simulink model "simu"  (R2023b)
settings: Solver=VariableStepAuto  StartTime=0.0  StopTime=8  RelTol=1e-3
libraries: simulink x6
settings Model: Creator=denis  LastModifiedBy=andre
settings OptimizationCC: ReuseModelBlockBuffer=off

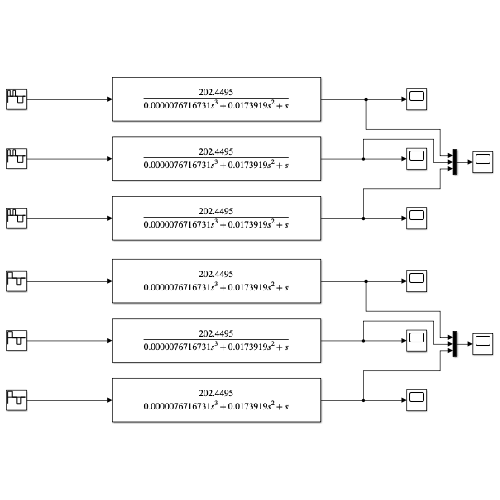
[thumbnail: Simulink's stored preview of the top-level diagram]
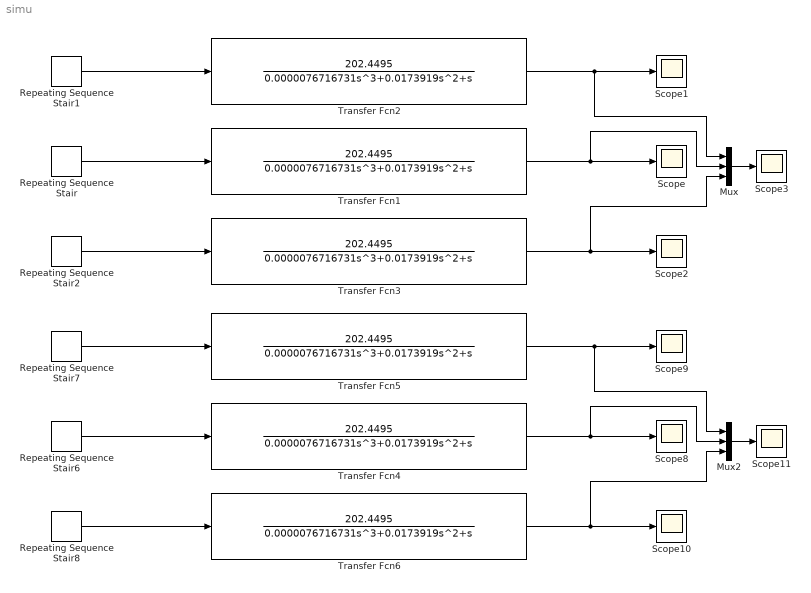
== system simu ==
  Mux : Mux  Inputs=3
  Mux2 : Mux  Inputs=3
  Repeating Sequence Stair : simulink/Sources/Repeating Sequence Stair  OutValues=7.5*[1 0 1 0 -1 -1 0].'  tsamp=1  OutMin=[]  OutMax=[]  OutDataTypeStr=double  OutputDataTypeScalingMode=double  OutDataType=fixdt(0,8)  ConRadixGroup=Best Precision: Vector-wise  OutScaling=2^-12
  Repeating Sequence Stair1 : simulink/Sources/Repeating Sequence Stair  OutValues=9*[1 0 1 0 -1 -1 0].'  tsamp=1  OutMin=[]  OutMax=[]  OutDataTypeStr=double  OutputDataTypeScalingMode=double  OutDataType=fixdt(0,8)  ConRadixGroup=Best Precision: Vector-wise  OutScaling=2^-12
  Repeating Sequence Stair2 : simulink/Sources/Repeating Sequence Stair  OutValues=6*[1 0 1 0 -1 -1 0].'  tsamp=1  OutMin=[]  OutMax=[]  OutDataTypeStr=double  OutputDataTypeScalingMode=double  OutDataType=fixdt(0,8)  ConRadixGroup=Best Precision: Vector-wise  OutScaling=2^-12
  Repeating Sequence Stair6 : simulink/Sources/Repeating Sequence Stair  OutValues=7.5*[1 0 -1 0].'  tsamp=1  OutMin=[]  OutMax=[]  OutDataTypeStr=double  OutputDataTypeScalingMode=double  OutDataType=fixdt(0,8)  ConRadixGroup=Best Precision: Vector-wise  OutScaling=2^-12
  Repeating Sequence Stair7 : simulink/Sources/Repeating Sequence Stair  OutValues=9*[1 0 -1 0].'  tsamp=1  OutMin=[]  OutMax=[]  OutDataTypeStr=double  OutputDataTypeScalingMode=double  OutDataType=fixdt(0,8)  ConRadixGroup=Best Precision: Vector-wise  OutScaling=2^-12
  Repeating Sequence Stair8 : simulink/Sources/Repeating Sequence Stair  OutValues=6*[1 0 -1 0].'  tsamp=1  OutMin=[]  OutMax=[]  OutDataTypeStr=double  OutputDataTypeScalingMode=double  OutDataType=fixdt(0,8)  ConRadixGroup=Best Precision: Vector-wise  OutScaling=2^-12
  Scope{,1..3,8..11} (8 alike) : Scope
  Transfer Fcn{1..6} (6 alike) : TransferFcn  Numerator=[202.4495]  Denominator=[0.0000076716731 0.0173919 1 0]
  wires:
  Repeating Sequence Stair/1 -> Transfer Fcn1/1
  Transfer Fcn1/1 -> Mux/2, Scope/1
  Transfer Fcn2/1 -> Mux/1, Scope1/1
  Repeating Sequence Stair1/1 -> Transfer Fcn2/1
  Transfer Fcn3/1 -> Mux/3, Scope2/1
  Repeating Sequence Stair2/1 -> Transfer Fcn3/1
  Mux/1 -> Scope3/1
  Mux2/1 -> Scope11/1
  Transfer Fcn5/1 -> Mux2/1, Scope9/1
  Transfer Fcn6/1 -> Mux2/3, Scope10/1
  Transfer Fcn4/1 -> Mux2/2, Scope8/1
  Repeating Sequence Stair8/1 -> Transfer Fcn6/1
  Repeating Sequence Stair6/1 -> Transfer Fcn4/1
  Repeating Sequence Stair7/1 -> Transfer Fcn5/1
